simulink model "simulacao_test1"  (R2018a)
settings: Solver=VariableStepAuto  StartTime=0.0  StopTime=10.0  RelTol=1e-3
settings Model: Creator=LabT5  LastModifiedBy=LabT5

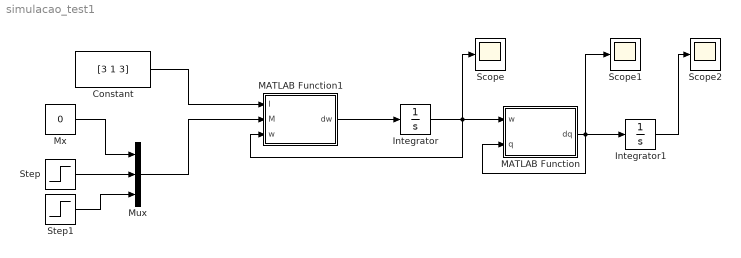
== system simulacao_test1 ==
  Constant : Constant  Value=[3 1 3]
  Integrator : Integrator
  Integrator1 : Integrator
  MATLAB Function : MATLAB Function  TreatAsAtomicUnit=on
  MATLAB Function1 : MATLAB Function  TreatAsAtomicUnit=on
  Mux : Mux  Inputs=3
  Mx : Constant  Value=0
  Scope : Scope
  Scope1 : Scope
  Scope2 : Scope
  Step : Step  After=-1  SampleTime=0
  Step1 : Step  After=-1  SampleTime=0
  wires:
  MATLAB Function1/1(dw) -> Integrator/1
  Integrator/1 -> Scope/1, MATLAB Function1/3(w), MATLAB Function/1(w)
  MATLAB Function/1(dq) -> Scope1/1, Integrator1/1, MATLAB Function/2(q)
  Integrator1/1 -> Scope2/1
  Mux/1 -> MATLAB Function1/2(M)
  Constant/1 -> MATLAB Function1/1(I)
  Mx/1 -> Mux/1
  Step/1 -> Mux/2
  Step1/1 -> Mux/3

== matlab function simulacao_test1/MATLAB Function1 ==
  data: I input; dw output; M input; w input
function dw = Eq_Euler(I,M,w)
wx = w(1);
wy = w(2);
wz = w(3);
Ix = I(1);
Iy = I(2);
Iz = I(3);

Mx = M(1);
My = M(2);
Mz = M(3);

dwx = (Mx - wy*wz*(Iz - Iy))/Ix;
dwy = (My - wx*wz*(Ix - Iz))/Iy;
dwz = (Mz - wx*wy*(Iy - Ix))/Iz;

dw=[dwx dwy dwz]';

== matlab function simulacao_test1/MATLAB Function ==
  data: w input; dq output; q input
function dq = cinematica(w,q)
%#eml
wx = w(1);
wy = w(2);
wz = w(3);

q = q/norm(q);
qteta = q(1);
qx = q(2);
qy = q(3);
qz = q(4);

W = [0 -wx -wy -wz; wx 0 wz -wy; wy -wz 0 wx; wz wy -wx 0];
dq=0.5*W*[qteta qx qy qz]';
